simulink model "ex3"  (R2020a)
settings: Solver=VariableStepAuto  StartTime=0.0  StopTime=10.0  RelTol=1e-3

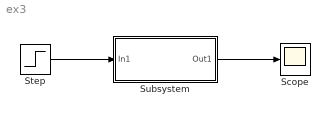
== system ex3 ==
  Scope : Scope
  Step : Step  SampleTime=0
  Subsystem : Subsystem  mask{R=10000, L=100, C=0.0001}
      mask prompts: R "R="; L "L="; C "C="
  wires:
  Step/1 -> Subsystem/1(In1)
  Subsystem/1(Out1) -> Scope/1

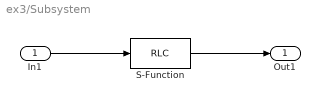
== system ex3/Subsystem ==
  In1 : Inport
  S-Function : S-Function  FunctionName=RLC  Parameters=A,B,C  SFunctionDeploymentMode=off  EnableBusSupport=off  mask{A=[-R/C -1/L;1/C 0], B=[1/L;0], C=[0 1]}
      mask prompts: A "A="; B "B="; C "C="
  Out1 : Outport
  wires:
  In1/1 -> S-Function/1
  S-Function/1 -> Out1/1
